simulink model "MLS4_4_rounded_step_inputR2024a"  (R2025b)
settings: Solver=FixedStepAuto  StartTime=0.0  StopTime=5  FixedStep=0.01  RelTol=1e-3
values from neighbouring files (symbols this model uses):
  st0 = 1.0    (= 1)    [Simulink_initial.m]    (also in initialize_simulink.m)
settings Model: Creator=Nico  LastModifiedBy=dixiao

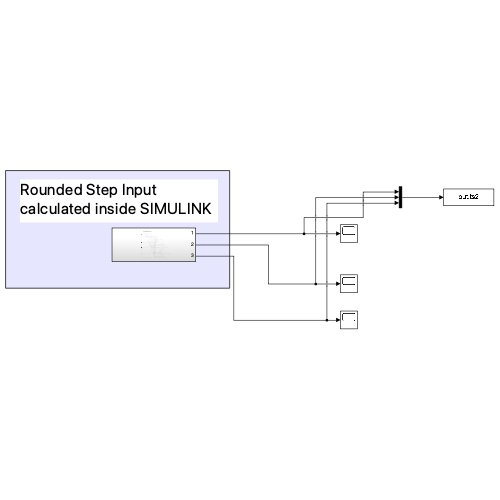
[thumbnail: Simulink's stored preview of the top-level diagram]
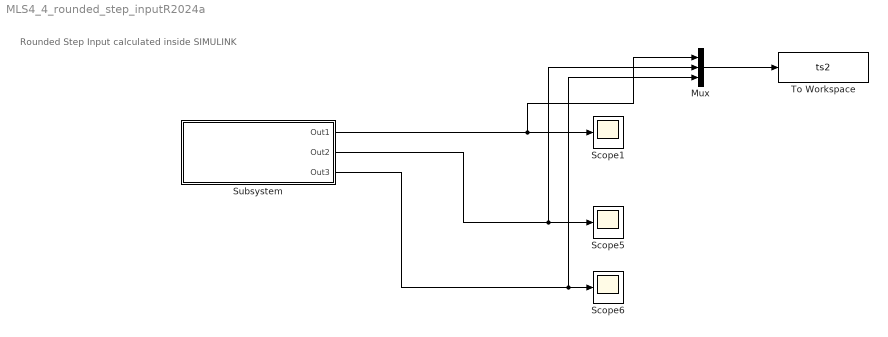
== system MLS4_4_rounded_step_inputR2024a ==
  note: Rounded Step Input
      | calculated inside SIMULINK
  Mux : Mux  Inputs=3
  Scope1 : Scope
      settings: ActiveDisplayYMinimum=-0.125  ActiveDisplayYMaximum=1.125
  Scope5 : Scope
      settings: ActiveDisplayYMinimum=-0.41667  ActiveDisplayYMaximum=3.75  DataLoggingVariableName=ScopeData2
  Scope6 : Scope
      settings: ActiveDisplayYMinimum=-34.753148536857786  ActiveDisplayYMaximum=40.218506159815369  DataLoggingVariableName=ScopeData3
  Subsystem : Subsystem
  To Workspace : ToWorkspace  VariableName=ts2  SaveFormat=Timeseries  SampleTime=-1
  wires:
  Subsystem/1(Out1) -> Mux/1, Scope1/1
  Subsystem/2(Out2) -> Mux/2, Scope5/1
  Subsystem/3(Out3) -> Mux/3, Scope6/1
  Mux/1 -> To Workspace/1

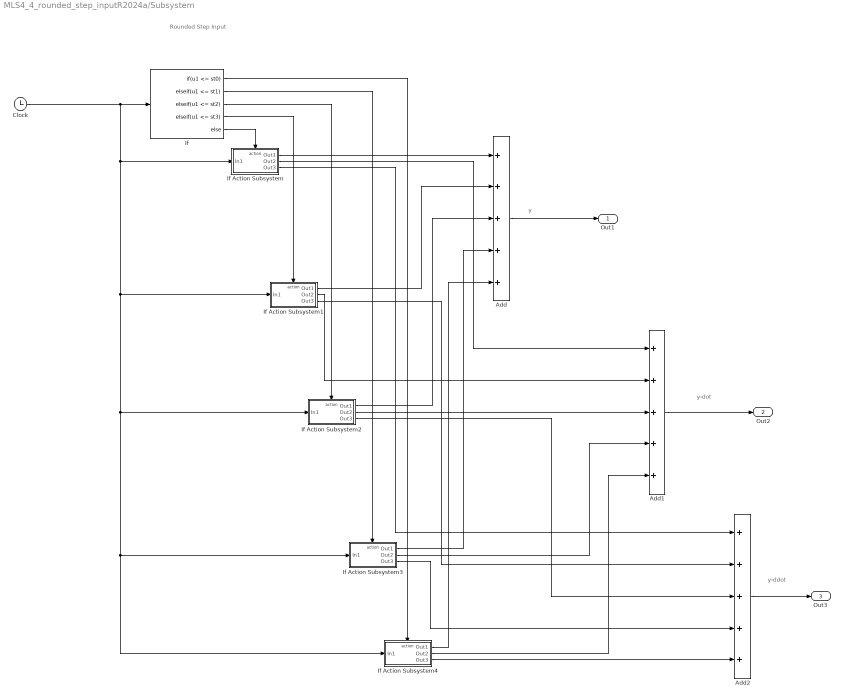
== system MLS4_4_rounded_step_inputR2024a/Subsystem ==
  note: Rounded Step Input
  note: y-ddot
  note: y-dot
  note: y
  Add : Sum  Inputs=+++++
  Add1 : Sum  Inputs=+++++
  Add2 : Sum  Inputs=+++++
  Clock : Clock
  If : If  IfExpression=u1 <= st0  ElseIfExpressions=u1 <= st1, u1 <= st2, u1 <= st3
  If Action Subsystem : Subsystem  TreatAsAtomicUnit=on
  If Action Subsystem1 : Subsystem  TreatAsAtomicUnit=on
  If Action Subsystem2 : Subsystem  TreatAsAtomicUnit=on
  If Action Subsystem3 : Subsystem  TreatAsAtomicUnit=on
  If Action Subsystem4 : Subsystem  TreatAsAtomicUnit=on
  Out1 : Outport
  Out2 : Outport  Port=2
  Out3 : Outport  Port=3
  wires:
  If Action Subsystem1/1(Out1) -> Add/2
  If/5 -> If Action Subsystem/Action
  If/3 -> If Action Subsystem2/Action
  If/2 -> If Action Subsystem3/Action
  If Action Subsystem/1(Out1) -> Add/1
  If Action Subsystem4/1(Out1) -> Add/5
  If/4 -> If Action Subsystem1/Action
  If/1 -> If Action Subsystem4/Action
  If Action Subsystem3/1(Out1) -> Add/4
  If Action Subsystem2/1(Out1) -> Add/3
  Add/1 -> Out1/1
  Add1/1 -> Out2/1
  Add2/1 -> Out3/1
  Clock/1 -> If Action Subsystem4/1(In1), If Action Subsystem3/1(In1), If Action Subsystem2/1(In1), If Action Subsystem1/1(In1), If Action Subsystem/1(In1), If/1
  If Action Subsystem/2(Out2) -> Add1/1
  If Action Subsystem/3(Out3) -> Add2/1
  If Action Subsystem1/2(Out2) -> Add1/2
  If Action Subsystem1/3(Out3) -> Add2/2
  If Action Subsystem2/2(Out2) -> Add1/3
  If Action Subsystem2/3(Out3) -> Add2/3
  If Action Subsystem3/3(Out3) -> Add2/4
  If Action Subsystem3/2(Out2) -> Add1/4
  If Action Subsystem4/2(Out2) -> Add1/5
  If Action Subsystem4/3(Out3) -> Add2/5

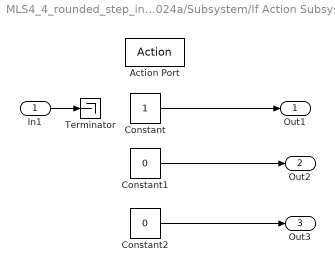
== system MLS4_4_rounded_step_inputR2024a/Subsystem/If Action Subsystem ==
  In1 : Inport
  Action Port : ActionPort  ActionPortLabel=else
  Constant : Constant
  Constant1 : Constant  Value=0
  Constant2 : Constant  Value=0
  Terminator : Terminator
  Out1 : Outport  OutputWhenDisabled=reset  InitialOutput=0
  Out2 : Outport  Port=2  OutputWhenDisabled=reset  InitialOutput=0
  Out3 : Outport  Port=3
  wires:
  Constant/1 -> Out1/1
  In1/1 -> Terminator/1
  Constant1/1 -> Out2/1
  Constant2/1 -> Out3/1

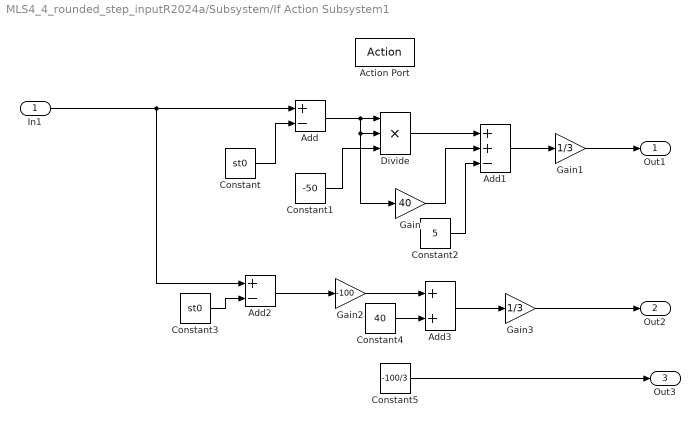
== system MLS4_4_rounded_step_inputR2024a/Subsystem/If Action Subsystem1 ==
  In1 : Inport
  Action Port : ActionPort  ActionPortLabel=elseif( u1 <= st3)
  Add : Sum  Inputs=+-
  Add1 : Sum  Inputs=++-
  Add2 : Sum  Inputs=+-
  Add3 : Sum
  Constant : Constant  Value=st0
  Constant1 : Constant  Value=-50
  Constant2 : Constant  Value=5
  Constant3 : Constant  Value=st0
  Constant4 : Constant  Value=40
  Constant5 : Constant  Value=-100/3
  Divide : Product  Inputs=***
  Gain : Gain  Gain=40
  Gain1 : Gain  Gain=1/3
  Gain2 : Gain  Gain=-100
  Gain3 : Gain  Gain=1/3
  Out1 : Outport  OutputWhenDisabled=reset  InitialOutput=0
  Out2 : Outport  Port=2  OutputWhenDisabled=reset  InitialOutput=0
  Out3 : Outport  Port=3  OutputWhenDisabled=reset  InitialOutput=0
  wires:
  In1/1 -> Add2/1, Add/1
  Constant1/1 -> Divide/3
  Constant/1 -> Add/2
  Add/1 -> Gain/1, Divide/2, Divide/1
  Divide/1 -> Add1/1
  Gain/1 -> Add1/2
  Constant2/1 -> Add1/3
  Add1/1 -> Gain1/1
  Gain1/1 -> Out1/1
  Add2/1 -> Gain2/1
  Gain2/1 -> Add3/1
  Add3/1 -> Gain3/1
  Constant3/1 -> Add2/2
  Constant4/1 -> Add3/2
  Gain3/1 -> Out2/1
  Constant5/1 -> Out3/1

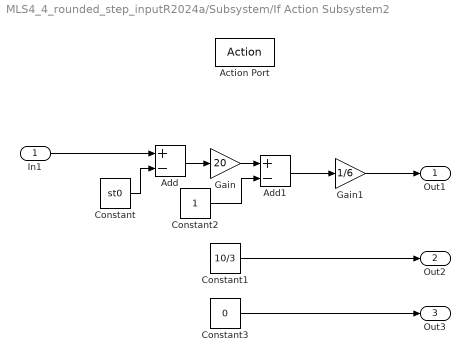
== system MLS4_4_rounded_step_inputR2024a/Subsystem/If Action Subsystem2 ==
  In1 : Inport
  Action Port : ActionPort  ActionPortLabel=elseif( u1 <= st2)
  Add : Sum  Inputs=+-
  Add1 : Sum  Inputs=+-
  Constant : Constant  Value=st0
  Constant1 : Constant  Value=10/3
  Constant2 : Constant
  Constant3 : Constant  Value=0
  Gain : Gain  Gain=20
  Gain1 : Gain  Gain=1/6
  Out1 : Outport  OutputWhenDisabled=reset  InitialOutput=0
  Out2 : Outport  Port=2  OutputWhenDisabled=reset  InitialOutput=0
  Out3 : Outport  Port=3  OutputWhenDisabled=reset  InitialOutput=0
  wires:
  In1/1 -> Add/1
  Constant/1 -> Add/2
  Add/1 -> Gain/1
  Gain/1 -> Add1/1
  Constant2/1 -> Add1/2
  Add1/1 -> Gain1/1
  Gain1/1 -> Out1/1
  Constant1/1 -> Out2/1
  Constant3/1 -> Out3/1

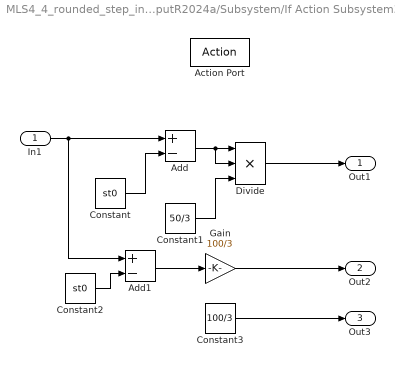
== system MLS4_4_rounded_step_inputR2024a/Subsystem/If Action Subsystem3 ==
  In1 : Inport
  Action Port : ActionPort  ActionPortLabel=elseif(u1 <= st1)
  Add : Sum  Inputs=+-
  Add1 : Sum  Inputs=+-
  Constant : Constant  Value=st0
  Constant1 : Constant  Value=50/3
  Constant2 : Constant  Value=st0
  Constant3 : Constant  Value=100/3
  Divide : Product  Inputs=***
  Gain : Gain  Gain=100/3
  Out1 : Outport  OutputWhenDisabled=reset  InitialOutput=0
  Out2 : Outport  Port=2  OutputWhenDisabled=reset  InitialOutput=0
  Out3 : Outport  Port=3  OutputWhenDisabled=reset  InitialOutput=0
  wires:
  In1/1 -> Add1/1, Add/1
  Constant/1 -> Add/2
  Add/1 -> Divide/2, Divide/1
  Constant1/1 -> Divide/3
  Divide/1 -> Out1/1
  Add1/1 -> Gain/1
  Constant2/1 -> Add1/2
  Gain/1 -> Out2/1
  Constant3/1 -> Out3/1

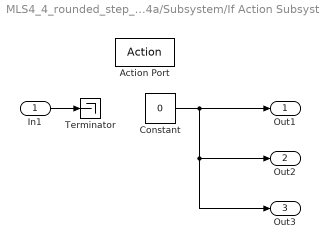
== system MLS4_4_rounded_step_inputR2024a/Subsystem/If Action Subsystem4 ==
  In1 : Inport
  Action Port : ActionPort  ActionPortLabel=if(u1 <= st0)
  Constant : Constant  Value=0
  Terminator : Terminator
  Out1 : Outport  OutputWhenDisabled=reset  InitialOutput=0
  Out2 : Outport  Port=2  OutputWhenDisabled=reset  InitialOutput=0
  Out3 : Outport  Port=3  OutputWhenDisabled=reset  InitialOutput=0
  wires:
  Constant/1 -> Out2/1, Out3/1, Out1/1
  In1/1 -> Terminator/1
